simulink library "lib_controls"  (Simulink 7.9)
settings: Solver=ode45  SolverMode=SingleTasking  StartTime=0.0  StopTime=10.0  RelTol=1e-3
undefined symbols (not defined in the file or in its folder): amb_tmp, cs_charge_deplete_bool, cs_charge_pwr, cs_charge_trq, cs_clt_tmp, cs_decel_fc_off, cs_decel_regen_threshold, cs_dl_assist_trq_threshold, cs_dl_regen_trq_threshold, cs_electric_decel_spd, cs_electric_launch_spd, cs_electric_launch_spd_hi, cs_electric_launch_spd_lo, cs_eng_min_spd, cs_eng_on_soc, cs_fc_init_state, cs_fc_max_pwr_frac, cs_fc_min_pwr_frac, cs_fc_on, cs_fc_pwr_opt, cs_fc_spd_opt, cs_fuzzy_fuel_mode, cs_hi_soc, cs_hi_trq_frac, cs_lo_soc, cs_lo_trq_frac, cs_max_gc_spd, cs_max_pwr, cs_max_pwr_fall_rate, cs_max_pwr_rise_rate, cs_mc_assist_max_frac, cs_mc_assist_min_frac, cs_mc_assist_slope, cs_mc_regen_max_frac, cs_mc_regen_min_frac, cs_mc_regen_slope, cs_mean_eff, cs_mean_eff_bool, cs_min_gc_spd, cs_min_off_time, cs_min_pwr, cs_min_trq_frac, cs_mph_avg_time, cs_off_trq_frac, cs_plot_output, cs_pwr, cs_regen_avg_time, cs_scale_factor, cs_shutoff, cs_soc_range, cs_spd, cs_target_soc, cs_trq_to_soc_factor, cvt_locus_pwr, cvt_locus_spd, cyc_mph, enable_sim_stop_distance, enable_sim_stop_max_spd, enable_sim_stop_speed, enable_sim_stop_time ... (+110)
libraries: lib_controls x124, simulink3 x13, simulink x5, lib_etc x1
(part 14 of 17)

== system lib_controls/<vc> series/gearbox control for series  HV and EV/shifting1 ==
  gear number : Inport
  Constant : Constant  Value=gb_shift_delay-1e-6
  Relational Operator : RelationalOperator  Operator=<  InputSameDT=on
  time since last shift : Subsystem
      mask Display: disp('time since\nlast shift')
  out_1 : Outport  InitialOutput=0
  wires:
  Relational Operator/1 -> out_1/1
  gear number/1 -> time since last shift/1(in_1)
  Constant/1 -> Relational Operator/2
  time since last shift/1(out_1) -> Relational Operator/1

== system lib_controls/<vc> series/gearbox control for series  HV and EV/upshift  command ==
  prev gear number : Inport
  engine load : Inport  Port=2
  engine speed : Inport  Port=3
  Mux : Mux  Inputs=2
  Relational Operator : RelationalOperator  Operator=<  InputSameDT=on
  load fraction : Subsystem  mask(Gear Selector){spd=gb_upshift_spd, load=gb_upshift_load}
      mask prompts: spd "Speeds:"; load "Load Fractions:"
      mask help:
      | This block will perform a linear interplation (extrapolation outside of bounds) to determine the shift point load fraction associated with the current gear number and speed.
      |
      | The Speeds parameter should be defined as an array of vectors containing speeds for each gear number.  The Load Fractions parameter should be defined as a array of vectors containing load fractions indexed by the speeds in the Speeds parameter for each gear number.
      mask Help:
      | Reference the base workspace variables - gb_**shift_spd and gb_**shift_load  where ** is either up for upshift conditions or dn for downshift conditions.
      | 
      | Or define the arrays as follows:
      | 
      | {[spd1 spd2 spd3 spd4]; [spd1 spd2 spd3 spd4]; ...}
      | 
      | {[load1 load2 load3 load4]; [load1 load2 load3 load4]; ...}
      | 
      | where each array contains one row for each gear in the gearbox.  Speeds should be defined in rad/s and loads as a decimal fraction.
  command : Outport  InitialOutput=0
  wires:
  load fraction/1(Out1) -> Relational Operator/2
  engine load/1 -> Relational Operator/1
  prev gear number/1 -> Mux/1
  Mux/1 -> load fraction/1(In1)
  engine speed/1 -> Mux/2
  Relational Operator/1 -> command/1

== system lib_controls/<vc> series/motor controller logic/Block NOTES ==
  note: This block models a motor/controller's logic, modulating the power input requirement as follows:
      | - enforcing the maximum current limit of the motor/controller
      | - shutting the motor off if the average speed over the time step ==0
      | - shutting the motor off if the transmission is shifting.

== system lib_controls/<vc> series/motor controller logic/Sign ==
  in_1 : Inport
  Constant : Constant  Value=0
  Relational Operator : RelationalOperator  Operator=>  InputSameDT=on
  Relational Operator1 : RelationalOperator  Operator=<  InputSameDT=on
  Sum : Sum  Inputs=+-  SaturateOnIntegerOverflow=on  InputSameDT=on  OutDataTypeStr=Inherit: Same as first input
  out_1 : Outport  InitialOutput=0
  wires:
  Sum/1 -> out_1/1
  Relational Operator/1 -> Sum/1
  Relational Operator1/1 -> Sum/2
  Constant/1 -> Relational Operator/2, Relational Operator1/2
  in_1/1 -> Relational Operator1/1, Relational Operator/1

== system lib_controls/<vc> series/series 'clutch' control/Block NOTES ==
  note: There is no clutch, per se, in the series hybrid vehicle, that is connected to
      | the engine.  This clutch control is provided to tell the fuel converter (a.k.a. engine)
      | when it can spin up freely.  The fuel converter spins up or down when the 'clutch' is
      | disengaged, and provides torque when the 'clutch' is engaged (signal==3).
      |
      | Here, the fuel converter spins up when the engine has been off within the
      | past 0.5 s (or one time step, whichever is greater).  At all other times, the fuel
      | converter provides torque to the generator.

== system lib_controls/Adaptive control strategy <cs>/Delta SOC expected from regen/Subsystem ==
  in_1 : Inport
  1/average time : Constant  Value=1/n
  Integrator : Integrator
  Product : Product  SaturateOnIntegerOverflow=on  RndMeth=Zero  InputSameDT=on  OutDataTypeStr=Inherit: Same as first input
  Sum : Sum  Inputs=+-  SaturateOnIntegerOverflow=on  InputSameDT=on  OutDataTypeStr=Inherit: Same as first input
  Transport Delay : TransportDelay  DelayTime=n
  out_1 : Outport  InitialOutput=0
  wires:
  1/average time/1 -> Product/2
  Product/1 -> out_1/1
  in_1/1 -> Integrator/1
  Sum/1 -> Product/1
  Transport Delay/1 -> Sum/2
  Integrator/1 -> Transport Delay/1, Sum/1

== system lib_controls/Adaptive control strategy <cs>/Finds operation  point - energy/emissions  weighting/Minimize the  energy used  and emissions ==
  note: Note: acc_elec_pwr_est is placed
      | outside of Min. Energy/emis due to the fact
      | that it is a FROM block. FROM blocks cannot
      | be placed inside of enabled sub-systems
  input vector : Inport
  "  1" : Constant  Value=0
  Demux : Demux  Outputs=8
  Logical Operator : Logic  Operator=NOT  Inputs=1
  Min. Energy/emis : Subsystem  TreatAsAtomicUnit=on
  Zero T/w/spd case : Subsystem
  Zero Treq or wreq case : Switch  Threshold=eps  SaturateOnIntegerOverflow=on  InputSameDT=on
  total fuel used (gal)1 : ToWorkspace  VariableName=cs_Impact
  Tfc : Outport
  wires:
  Logical Operator/1 -> Min. Energy/emis/Enable
  Demux/8 -> Min. Energy/emis/8(ess_tmp)
  Min. Energy/emis/2(Impact) -> total fuel used (gal)1/1
  Zero Treq or wreq case/1 -> Tfc/1
  "  1"/1 -> Zero Treq or wreq case/1
  Min. Energy/emis/1(Tfc) -> Zero Treq or wreq case/3
  Demux/1 -> Zero T/w/spd case/1(Treq), Min. Energy/emis/1(Treq)
  Demux/2 -> Zero T/w/spd case/2(wreq), Min. Energy/emis/2(wreq)
  Demux/7 -> Min. Energy/emis/7(ex_cat_tmp)
  Demux/6 -> Min. Energy/emis/6(fc_clt_tmp)
  Demux/5 -> Min. Energy/emis/5(cyc_mph_r)
  Demux/4 -> Min. Energy/emis/4(SOC)
  Demux/3 -> Min. Energy/emis/3(DeltaSOC regen)
  input vector/1 -> Demux/1
  Zero T/w/spd case/1(zero req flag) -> Zero Treq or wreq case/2, Logical Operator/1
  [acc_elec_pwr_est] -> Min. Energy/emis/9(Elect Aux  Load Power)

== system lib_controls/Adaptive control strategy <cs>/Finds operation  point - energy/emissions  weighting/Subsystem ==
  in_1 : Inport
  1/average time : Constant  Value=1/n
  Integrator : Integrator
  Product : Product  SaturateOnIntegerOverflow=on  RndMeth=Zero  InputSameDT=on  OutDataTypeStr=Inherit: Same as first input
  Sum : Sum  Inputs=+-  SaturateOnIntegerOverflow=on  InputSameDT=on  OutDataTypeStr=Inherit: Same as first input
  Transport Delay : TransportDelay  DelayTime=n
  out_1 : Outport  InitialOutput=0
  wires:
  1/average time/1 -> Product/2
  Product/1 -> out_1/1
  in_1/1 -> Integrator/1
  Sum/1 -> Product/1
  Transport Delay/1 -> Sum/2
  Integrator/1 -> Transport Delay/1, Sum/1

== system lib_controls/Fuzzy Logic control strategy <cs>/Fuzzy logic Code/Block NOTES ==
  note: This block calls the Fuzzy Controller through the Matlab-Function module.
      | The Fuzzy Control algorithm is written in MATLAB script. This makes it easy
      | for the user to edit the fuzzy algorithm and make changes.
      |
      | For more information on Matlab-functions, please refer to the MATLAB help files.

== system lib_controls/Fuzzy Logic control strategy <cs>/Input Scaling/Block NOTES ==
  note: INPUT SCALING
  note: In this block, inputs to the Fuzzy Logic controller are computed. The Current torque demand on the ICE
      | and the SoC are input as 2 scaled variables to the fuzzy controller. Both inputs are scaled from 1 to 11.
      |
      | For SoC, a value of cs_lo_soc would correspond to 1 and a value of cs_hi_soc would correspond to 11,
      | linearly interpolating between them.
      |
      | For the ICE Torque, any torque demand less than the target ICE torque would scale from 1 to 6. Any torque
      | demand greater than the target ICE torque would scale from 6 to 11 (the 2 being piecewise linear).
      |
      | The target ICE torque is the x g/s fuel use line, (FUEL USE MODE), or the peak efficiency line
      | (EFFICIENCY MODE).

== system lib_controls/Fuzzy Logic control strategy <cs>/Output scaling/Block NOTES ==
  note: OUTPUT SCALING
      | This bock scales the outputs of the controller to match the size of the components.
      | The scaling affects the way control signal is fed into the actuators. The scaling is done based
      | on the membership functions of the Fuzzy Control block.
      |
      | Here:
      |  DELTA ALPHA is scaled from 1 to 11, 1 representing zero torque, 6 representing target Torque
      | and 11 representing Max ICE torque. (the 2 regions being piecewise linear).

== system lib_controls/Fuzzy Logic control strategy with Emissions <cs>/Fuzzy logic Code/Block NOTES ==
  note: This block calls the Fuzzy Controller through the Matlab-Function module.
      | The Fuzzy Control algorithm is written in MATLAB script. This makes it easy
      | for the user to edit the fuzzy algorithm and make changes.
      |
      | For more information on Matlab-functions, please refer to the MATLAB help files.

== system lib_controls/Fuzzy Logic control strategy with Emissions <cs>/Input Scaling/Block NOTES ==
  note: In this block, inputs to the Fuzzy Logic controller are computed. The Current torque demand on the ICE
      | and the SoC are input as 2 scaled variables to the fuzzy controller. Both inputs are scaled from 1 to 11.
      |
      | For SoC, a value of cs_lo_soc would correspond to 1 and a value of cs_hi_soc would correspond to 11,
      | linearly interpolating between them.
      |
      | For the ICE Torque, any torque demand less than the target ICE torque would scale from 1 to 6. Any torque
      | demand greater than the target ICE torque would scale from 6 to 11 (the 2 being piecewise linear).
  note: INPUT SCALING
  note: TARGET TORQUE COMPUTATION
  note: The target (optimal) torque for a particular speed requested from the ICE is calculated using a weighted average of
      | the efficiency and emissions data for a particular speed in consideration.
      |
      | The calculation of the target torque involves calculating the minimum of a cost function. The competing quantities
      | of the cost function include the emissions and fuel economy for all torques at that speed, weighed by their
      | respective weights.
      |
      | The relative importance for the competing quantities (weights) are changed during the simulation,
      | to reflect changes in driving conditions. For example, during a cold start, emissions are given higher priority. Also,
      | if the electric motor has been reaching it's maximum assist capability in the wake of the torque request not being met,
      | then emissions are sacrificed for higher torque from the ICE.

== system lib_controls/Fuzzy Logic control strategy with Emissions <cs>/Output scaling/Block NOTES ==
  note: OUTPUT SCALING
      | This bock scales the outputs of the controller to match the size of the components.
      | The scaling affects the way control signal is fed into the actuators. The scaling is done based
      | on the membership functions of the Fuzzy Control block.
      |
      | Here:
      |  DELTA ALPHA is scaled from 1 to 11, 1 representing zero torque, 6 representing target Torque
      | and 11 representing Max ICE torque. (the 2 regions being piecewise linear).

== system lib_controls/Fuzzy Logic control strategy with Emissions <cs>/SoC /Block NOTES ==
  note: This block scales the battery SOC so as to feed it into the Fuzzy controller.
      | 1 represents the lower limit of allowable battery SOC while 11 represents the higher
      | limit of allowable battery SOC.

== system lib_controls/Insight electric assist control strategy <cs> DIRECT SPLIT/Alternator Function/Block NOTES ==
  note: ALTERNATOR FUNCTION
      | In the HONDA Insight, there is no separate alternator for the vehicle in the powertrain
      | to supply power for the accessory loads. The main electric motor is the alternator for the vehicle.
      | Thus, it always produces a small negative torque for driving the accessory loads.  But the electric
      | motor has to take into account, the component efficiencies, and thus, is forced
      | to regenerate a little more than the accessory load.
      |
      | During assist, the battery pack supplies the electrical accessory loads.

== system lib_controls/Insight electric assist control strategy <cs> DIRECT SPLIT/SoC Correction/Block NOTES ==
  note: HONDA INSIGHT SoC Correction STRATEGY
      |
      | In the HONDA Insight strategy, the electric motor assist is independent on the SoC of the battery pack
      | except at low and high SoCs. (Based on test results).
      |
      | At high SoCs, above 0.8, all regeneration (charging) is stopped. At low SoCs, below 0.35 (approx),
      | the assist capacity of the motor is limited, and all assist is cut off below an SoC of 0.2.

== system lib_controls/SubSystem/braking strategy/Block NOTES ==
  note: This controller determines how much braking
      | force the front and rear  friction brakes will supply.

== system lib_controls/SubSystem/front and rear brake controller (achievable)/Block NOTES ==
  note: This block apportions required friction braking force between the
      | front (drive) and rear brakes.  Vehicle speed for brake strategy is
      | computed assuming zero slip.

== system lib_controls/SubSystem/front and rear brake controller (achievable)/braking force supplied by front friction brakes (N) ==
  add'l braking force req'd (N) : Inport
  possible speed (mph) : Inport  Port=2
  max front brake force (N) : Inport  Port=3
  Block NOTES : Subsystem
      mask Display: disp('Block\nNOTES')
  Constant : Constant  Value=1+eps
  Constant1 : Constant  Value=0.6
  Keep 0<frac<1 : Saturate  UpperLimit=1  LowerLimit=0
  MinMax : MinMax  Function=max  Inputs=2  SaturateOnIntegerOverflow=on  InputSameDT=on
  Product : Product  Inputs=**  SaturateOnIntegerOverflow=on  RndMeth=Zero  InputSameDT=on  OutDataTypeStr=Inherit: Same as first input
  Product1 : Product  Inputs=*/  SaturateOnIntegerOverflow=on  RndMeth=Zero  InputSameDT=on  OutDataTypeStr=Inherit: Same as first input
  Saturation : Saturate  UpperLimit=max(wh_fa_fric_brake_mph)  LowerLimit=min(wh_fa_fric_brake_mph)
  Saturation1 : Saturate  UpperLimit=max(wh_fa_dl_brake_mph)  LowerLimit=min(wh_fa_dl_brake_mph)
  Sum : Sum  Inputs=-+  SaturateOnIntegerOverflow=on  InputSameDT=on  OutDataTypeStr=Inherit: Same as first input
  Switch1 : Switch  Threshold=eps  SaturateOnIntegerOverflow=on  InputSameDT=on
  driveline braking fraction : Lookup  InputValues=wh_fa_dl_brake_mph  Table=wh_fa_dl_brake_frac  SaturateOnIntegerOverflow=on
  front friction braking fraction : Lookup  InputValues=wh_fa_fric_brake_mph  Table=wh_fa_fric_brake_frac  SaturateOnIntegerOverflow=on
  braking force from front-axle friction brakes (N) : Outport  InitialOutput=0
  wires:
  Keep 0<frac<1/1 -> Product/2
  Switch1/1 -> Keep 0<frac<1/1
  MinMax/1 -> braking force from front-axle friction brakes (N)/1
  Product/1 -> MinMax/1
  max front brake force (N)/1 -> MinMax/2
  add'l braking force req'd (N)/1 -> Product/1
  Constant/1 -> Sum/2
  driveline braking fraction/1 -> Sum/1
  front friction braking fraction/1 -> Product1/1
  Product1/1 -> Switch1/1
  Sum/1 -> Product1/2, Switch1/2
  Constant1/1 -> Switch1/3
  Saturation/1 -> front friction braking fraction/1
  Saturation1/1 -> driveline braking fraction/1
  possible speed (mph)/1 -> Saturation1/1, Saturation/1

== system lib_controls/SubSystem/shifting/time since last shift ==
  in_1 : Inport
  just shifted : Subsystem
      mask Display: disp('just\nshifted')
  timer : Subsystem
      mask Display: disp('timer')
  out_1 : Outport  InitialOutput=0
  wires:
  in_1/1 -> just shifted/1(in_1)
  just shifted/1(out_1) -> timer/1(trigger)
  timer/1(time) -> out_1/1

== system lib_controls/SubSystem/sim stop subsystem/Block NOTES ==
  note: This block controls the simulation stop time.  The simulation maybe
      | stop based on the achievement of a specified speed, a max speed, a time, a distance, or an engine condition.

== system lib_controls/SubSystem/sim stop subsystem/stop sim distance ==
  distance : Inport
  Enable : EnablePort
  Const : Constant  Value=sim_stop_distance
  Relational Operator2 : RelationalOperator  Operator=>  InputSameDT=on
  Out1 : Outport  InitialOutput=0
  wires:
  distance/1 -> Relational Operator2/1
  Const/1 -> Relational Operator2/2
  Relational Operator2/1 -> Out1/1

== system lib_controls/SubSystem/sim stop subsystem/stop sim fc ==
  engine on? : Inport
  Enable : EnablePort
  Clock : Clock
  Const : Constant  Value=j17_endtimes
  Logical Operator : Logic
  Logical Operator1 : Logic  Operator=OR
  Logical Operator2 : Logic  Operator=OR  Inputs=1
  Manual Switch : simulink3/Nonlinear/Manual Switch  sw=0  action=0
  Memory : Memory
  Relational Operator : RelationalOperator  Operator===  InputSameDT=on
  Relational Operator1 : RelationalOperator  InputSameDT=on
  Out1 : Outport  InitialOutput=0
  wires:
  Manual Switch/1 -> Logical Operator2/1
  Relational Operator1/1 -> Manual Switch/2
  Relational Operator/1 -> Manual Switch/1
  Clock/1 -> Relational Operator1/1, Relational Operator/1
  Const/1 -> Relational Operator1/2, Relational Operator/2
  engine on?/1 -> Logical Operator1/1
  Memory/1 -> Logical Operator1/2
  Logical Operator1/1 -> Memory/1, Logical Operator/1
  Logical Operator2/1 -> Logical Operator/2
  Logical Operator/1 -> Out1/1

== system lib_controls/SubSystem/sim stop subsystem/stop sim max spd ==
  speed : Inport
  Enable : EnablePort
  Block NOTES : Subsystem
      mask Display: disp('Block\nNOTES')
  Const : Constant  Value=eps
  Logical Operator : Logic
  Relational Operator2 : RelationalOperator  Operator=>  InputSameDT=on
  Relational Operator3 : RelationalOperator  Operator=<=  InputSameDT=on
  Transport Delay : TransportDelay  DelayTime=(gb_shift_delay*5)+1
  Out1 : Outport  InitialOutput=0
  wires:
  Const/1 -> Relational Operator2/2
  Relational Operator2/1 -> Logical Operator/2
  Logical Operator/1 -> Out1/1
  speed/1 -> Relational Operator3/1, Relational Operator2/1, Transport Delay/1
  Transport Delay/1 -> Relational Operator3/2
  Relational Operator3/1 -> Logical Operator/1

== system lib_controls/SubSystem/sim stop subsystem/stop sim speed ==
  speed : Inport
  Enable : EnablePort
  Const : Constant  Value=sim_stop_speed
  Relational Operator2 : RelationalOperator  Operator=>  InputSameDT=on
  Out1 : Outport  InitialOutput=0
  wires:
  Relational Operator2/1 -> Out1/1
  Const/1 -> Relational Operator2/2
  speed/1 -> Relational Operator2/1

== system lib_controls/SubSystem/sim stop subsystem/stop sim time ==
  time : Inport
  Enable : EnablePort
  Const : Constant  Value=sim_stop_time
  Relational Operator2 : RelationalOperator  Operator=>  InputSameDT=on
  Out1 : Outport  InitialOutput=0
  wires:
  time/1 -> Relational Operator2/1
  Const/1 -> Relational Operator2/2
  Relational Operator2/1 -> Out1/1

== system lib_controls/SubSystem/traction control/Block NOTES ==
  note: Requested speed and force are limited by the
      | tractive characteristics of the tires in this block.

== system lib_controls/SubSystem/traction control/apply tire traction limit to req'd speed (m/s) ==
  "requested time-step  average vehicle speed (m/s) " : Inport
  vehicle speed at beginning of time step (m/s) : Inport  Port=2
  Block NOTES : Subsystem
      mask Display: disp('Block\nNOTES')
  Clock : Clock
  Constant : Constant  Value=veh_gravity
  Constant1 : Constant  Value=0.5*veh_gravity*wh_2nd_rrc
  Constant10 : Constant  Value=veh_gravity
  Constant11 : Constant  Value=wh_1st_rrc
  Constant2 : Constant  Value=max(wh_slip_force_coeff)*veh_gravity*veh_front_wt_frac
  Constant3 : Constant  Value=0.125*veh_air_density*veh_CD*veh_FA
  Constant4 : Constant  Value=max(wh_slip_force_coeff)*veh_cg_height/veh_wheelbase
  Constant6 : Constant  Value=0.375*veh_air_density*veh_CD*veh_FA
  Constant7 : Constant  Value=0.5*veh_gravity*wh_2nd_rrc
  Constant9 : Constant  Value=max(wh_slip_force_coeff)*veh_cg_height/veh_wheelbase
  Fcn : Fcn  Expr=1/u
  Memory : Memory  X0=-0.1
  MinMax : MinMax  Inputs=2  SaturateOnIntegerOverflow=on  InputSameDT=on
  Product : Product  Inputs=4  SaturateOnIntegerOverflow=on  RndMeth=Zero  InputSameDT=on  OutDataTypeStr=Inherit: Same as first input
  Product{1,3,6..7,9..11} (7 alike) : Product  Inputs=3  SaturateOnIntegerOverflow=on  RndMeth=Zero  InputSameDT=on  OutDataTypeStr=Inherit: Same as first input
  Product2 : Product  Inputs=4  SaturateOnIntegerOverflow=on  RndMeth=Zero  InputSameDT=on  OutDataTypeStr=Inherit: Same as first input
  Product4 : Product  SaturateOnIntegerOverflow=on  RndMeth=Zero  InputSameDT=on  OutDataTypeStr=Inherit: Same as first input
  Product5 : Product  SaturateOnIntegerOverflow=on  RndMeth=Zero  InputSameDT=on  OutDataTypeStr=Inherit: Same as first input
  Product8 : Product  SaturateOnIntegerOverflow=on  RndMeth=Zero  InputSameDT=on  OutDataTypeStr=Inherit: Same as first input
  Sum : Sum  Inputs=+---+-+  SaturateOnIntegerOverflow=on  InputSameDT=on  OutDataTypeStr=Inherit: Same as first input
  Sum1 : Sum  Inputs=+-  SaturateOnIntegerOverflow=on  InputSameDT=on  OutDataTypeStr=Inherit: Same as first input
  Sum2 : Sum  Inputs=++++  SaturateOnIntegerOverflow=on  InputSameDT=on  OutDataTypeStr=Inherit: Same as first input
  Sum3 : Sum  Inputs=-----+  SaturateOnIntegerOverflow=on  InputSameDT=on  OutDataTypeStr=Inherit: Same as first input
  Sum4 : Sum  SaturateOnIntegerOverflow=on  InputSameDT=on  OutDataTypeStr=Inherit: Same as first input
  Sum5 : Sum  SaturateOnIntegerOverflow=on  InputSameDT=on  OutDataTypeStr=Inherit: Same as first input
  Sum6 : Sum  SaturateOnIntegerOverflow=on  InputSameDT=on  OutDataTypeStr=Inherit: Same as first input
  Sum7 : Sum  Inputs=+++-  SaturateOnIntegerOverflow=on  InputSameDT=on  OutDataTypeStr=Inherit: Same as first input
  Trig Fn4 : Trigonometry  Operator=cos
  Trig Fn : Trigonometry  Operator=atan
  Trig Fn1 : Trigonometry
  current veh mass (kg){,1..7} (8 alike) : lib_controls/SubSystem/current veh mass (kg)
      settings: RTWFcnNameOpts=Auto  RTWFileNameOpts=Auto
  max speed at END of time step given tire traction limit (m/s) : Subsystem
      mask Display: disp('/')
  max time-step average speed (m/s) : Gain  Gain=0.5  SaturateOnIntegerOverflow=on  OutDataTypeStr=Inherit: Same as input  ParamDataTypeStr=Inherit: Same as input
  min speed at END of time step given tire traction limit (m/s) : Subsystem
      mask Display: disp('/')
  min time-step average speed (m/s) : Gain  Gain=0.5  SaturateOnIntegerOverflow=on  OutDataTypeStr=Inherit: Same as input  ParamDataTypeStr=Inherit: Same as input
  requested time-step average speed limited by tire traction (m/s) : MinMax  Function=max  Inputs=2  SaturateOnIntegerOverflow=on  InputSameDT=on
  out_1 : Outport  InitialOutput=0
  wires:
  current veh mass (kg)7/1 -> Product6/3
  current veh mass (kg)5/1 -> Product7/3
  current veh mass (kg)3/1 -> Product2/4
  current veh mass (kg)2/1 -> Product9/3
  current veh mass (kg)1/1 -> Product/4
  current veh mass (kg)/1 -> Product11/3
  Constant/1 -> Product11/1
  Product11/1 -> Sum3/2, Sum/2
  Sum6/1 -> Product11/2
  Trig Fn1/1 -> Product10/3, Sum6/2
  Constant10/1 -> Product10/2
  Constant4/1 -> Product10/1, Product2/1
  Product10/1 -> Sum/6
  Product3/1 -> Sum/7, Sum3/6
  current veh mass (kg)4/1 -> Product3/2
  max time-step average speed (m/s)/1 -> MinMax/2
  "requested time-step  average vehicle speed (m/s) "/1 -> MinMax/1
  Sum5/1 -> max time-step average speed (m/s)/1
  Constant2/1 -> Product9/1
  Constant11/1 -> Product8/1
  Product8/1 -> Sum6/1
  Trig Fn4/1 -> Product9/2, Product8/2, Product/3, Product7/2
  Clock/1 -> Memory/1, Sum1/1
  Sum1/1 -> Fcn/1
  Memory/1 -> Sum1/2
  current veh mass (kg)6/1 -> Product5/1
  Sum2/1 -> max speed at END of time step given tire traction limit (m/s)/2(in_2)
  min time-step average speed (m/s)/1 -> requested time-step average speed limited by tire traction (m/s)/2
  requested time-step average speed limited by tire traction (m/s)/1 -> out_1/1
  Sum4/1 -> min time-step average speed (m/s)/1
  min speed at END of time step given tire traction limit (m/s)/1(out_1) -> Sum4/1
  MinMax/1 -> requested time-step average speed limited by tire traction (m/s)/1
  Sum3/1 -> min speed at END of time step given tire traction limit (m/s)/1(in_1)
  Sum7/1 -> min speed at END of time step given tire traction limit (m/s)/2(in_2)
  Constant7/1 -> Product7/1
  Constant9/1 -> Product6/1
  Constant6/1 -> Product4/2
  Product4/1 -> Sum2/1, Sum7/1
  Product7/1 -> Sum2/2, Sum7/2
  Product5/1 -> Sum2/3, Sum7/3
  Product6/1 -> Sum2/4, Sum7/4
  Trig Fn/1 -> Trig Fn4/1, Trig Fn1/1
  vehicle speed at beginning of time step (m/s)/1 -> Sum5/2, Sum4/2, Product4/1, Product3/1, Product2/2, Product1/3, Product1/2, Product/2
  [grade] -> Trig Fn/1
  max speed at END of time step given tire traction limit (m/s)/1(out_1) -> Sum5/1
  Product2/1 -> Sum3/5, Sum/5
  Product9/1 -> Sum3/1, Sum/1
  Product/1 -> Sum3/3, Sum/3
  Product1/1 -> Sum3/4, Sum/4
  Sum/1 -> max speed at END of time step given tire traction limit (m/s)/1(in_1)
  Fcn/1 -> Product6/2, Product5/2, Product3/3, Product2/3
  Constant3/1 -> Product1/1
  Constant1/1 -> Product/1

== system lib_controls/SubSystem/traction control/enforce max.  front axle tractive force  due to slip (N) ==
  tractive force req'd at tire/road interface (N) : Inport
  requested time-step average vehicle speed (m/s) : Inport  Port=2
  speed at beginning of time step (m/s) : Inport  Port=3
  " " : MinMax  Inputs=2  SaturateOnIntegerOverflow=on  InputSameDT=on
  Block NOTES : Subsystem
      mask Display: disp('Block\nNOTES')
  Clock : Clock
  Constant : Constant  Value=veh_cg_height/veh_wheelbase
  Constant1 : Constant  Value=veh_gravity*veh_front_wt_frac
  Constant2 : Constant  Value=max(wh_slip_force_coeff)
  Gain : Gain  Gain=-1  SaturateOnIntegerOverflow=on  OutDataTypeStr=Inherit: Same as input  ParamDataTypeStr=Inherit: Same as input
  Gain1 : Gain  Gain=2  SaturateOnIntegerOverflow=on  OutDataTypeStr=Inherit: Same as input  ParamDataTypeStr=Inherit: Same as input
  Gain2 : Gain  Gain=veh_gravity  SaturateOnIntegerOverflow=on  OutDataTypeStr=Inherit: Same as input  ParamDataTypeStr=Inherit: Same as input
  Memory1 : Memory  X0=-0.1
  Product : Product  Inputs=*/  SaturateOnIntegerOverflow=on  RndMeth=Zero  InputSameDT=on  OutDataTypeStr=Inherit: Same as first input
  Product1 : Product  Inputs=3  SaturateOnIntegerOverflow=on  RndMeth=Zero  InputSameDT=on  OutDataTypeStr=Inherit: Same as first input
  Product2 : Product  SaturateOnIntegerOverflow=on  RndMeth=Zero  InputSameDT=on  OutDataTypeStr=Inherit: Same as first input
  Product3 : Product  Inputs=3  SaturateOnIntegerOverflow=on  RndMeth=Zero  InputSameDT=on  OutDataTypeStr=Inherit: Same as first input
  Sum : Sum  Inputs=+-  SaturateOnIntegerOverflow=on  InputSameDT=on  OutDataTypeStr=Inherit: Same as first input
  Sum1 : Sum  Inputs=+-  SaturateOnIntegerOverflow=on  InputSameDT=on  OutDataTypeStr=Inherit: Same as first input
  Sum2 : Sum  SaturateOnIntegerOverflow=on  InputSameDT=on  OutDataTypeStr=Inherit: Same as first input
  Trig Fn : Trigonometry  Operator=atan
  Trig Fn1 : Trigonometry
  Trig Fn2 : Trigonometry  Operator=cos
  current veh mass (kg) : lib_controls/SubSystem/current veh mass (kg)
      settings: RTWFcnNameOpts=Auto  RTWFileNameOpts=Auto
  tractive force request limited by slip-threshhold force (N)1 : MinMax  Function=max  Inputs=2  SaturateOnIntegerOverflow=on  InputSameDT=on
  weight on front axle (N) : Sum  Inputs=-+  SaturateOnIntegerOverflow=on  InputSameDT=on  OutDataTypeStr=Inherit: Same as first input
  slip-limited force (N) : Outport  InitialOutput=0
  weight on front axle (N)1 : Outport  Port=2  InitialOutput=0
  wires:
  current veh mass (kg)/1 -> Product1/3, Product3/1
  Trig Fn2/1 -> Product3/2
  Constant1/1 -> Product3/3
  Product3/1 -> weight on front axle (N)/2
  Trig Fn/1 -> Trig Fn2/1, Trig Fn1/1
  Gain2/1 -> Sum2/2
  Trig Fn1/1 -> Gain2/1
  [grade] -> Trig Fn/1
  Sum2/1 -> Product1/2
  Gain1/1 -> Sum2/1
  tractive force request limited by slip-threshhold force (N)1/1 -> slip-limited force (N)/1
  " "/1 -> tractive force request limited by slip-threshhold force (N)1/1
  Product2/1 -> Gain/1, " "/1
  tractive force req'd at tire/road interface (N)/1 -> " "/2
  Constant2/1 -> Product2/2
  Gain/1 -> tractive force request limited by slip-threshhold force (N)1/2
  Product/1 -> Gain1/1
  Sum1/1 -> Product/2
  Memory1/1 -> Sum1/2
  Clock/1 -> Memory1/1, Sum1/1
  Sum/1 -> Product/1
  speed at beginning of time step (m/s)/1 -> Sum/2
  requested time-step average vehicle speed (m/s)/1 -> Sum/1
  weight on front axle (N)/1 -> weight on front axle (N)1/1, Product2/1
  Constant/1 -> Product1/1
  Product1/1 -> weight on front axle (N)/1

== system lib_controls/SubSystem/traction control 2 axle/Block NOTES ==
  note: Requested speed and force are limited by the
      | tractive characteristics of the tires in this block.

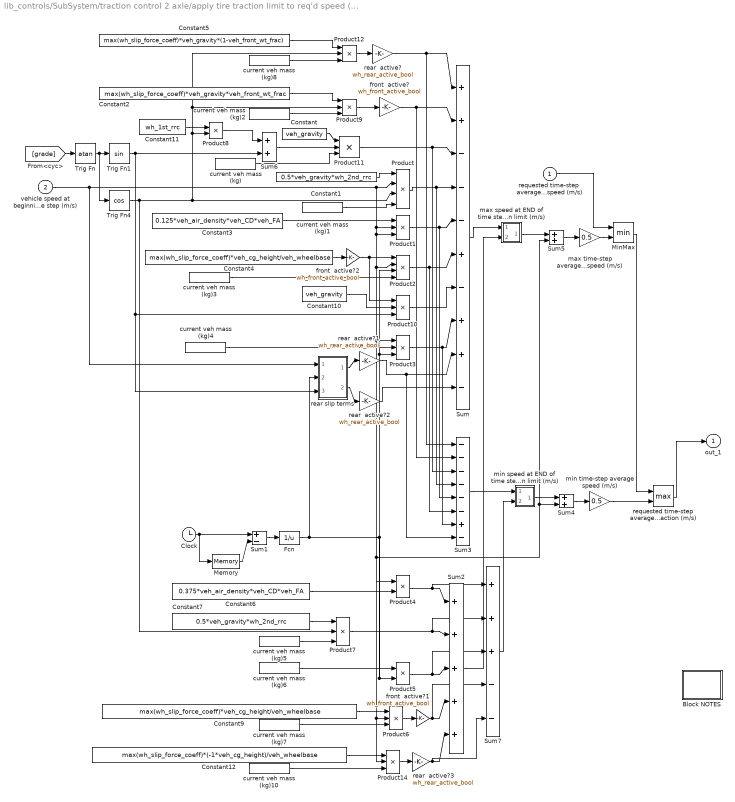
== system lib_controls/SubSystem/traction control 2 axle/apply tire traction limit to req'd speed (m/s) ==
  "requested time-step  average vehicle speed (m/s) " : Inport
  vehicle speed at beginning of time step (m/s) : Inport  Port=2
  Block NOTES : Subsystem
      mask Display: disp('Block\nNOTES')
  Clock : Clock
  Constant : Constant  Value=veh_gravity
  Constant1 : Constant  Value=0.5*veh_gravity*wh_2nd_rrc
  Constant10 : Constant  Value=veh_gravity
  Constant11 : Constant  Value=wh_1st_rrc
  Constant12 : Constant  Value=max(wh_slip_force_coeff)*(-1*veh_cg_height)/veh_wheelbase
  Constant2 : Constant  Value=max(wh_slip_force_coeff)*veh_gravity*veh_front_wt_frac
  Constant3 : Constant  Value=0.125*veh_air_density*veh_CD*veh_FA
  Constant4 : Constant  Value=max(wh_slip_force_coeff)*veh_cg_height/veh_wheelbase
  Constant5 : Constant  Value=max(wh_slip_force_coeff)*veh_gravity*(1-veh_front_wt_frac)
  Constant6 : Constant  Value=0.375*veh_air_density*veh_CD*veh_FA
  Constant7 : Constant  Value=0.5*veh_gravity*wh_2nd_rrc
  Constant9 : Constant  Value=max(wh_slip_force_coeff)*veh_cg_height/veh_wheelbase
  Fcn : Fcn  Expr=1/u
  Memory : Memory  X0=-0.1
  MinMax : MinMax  Inputs=2  SaturateOnIntegerOverflow=on  InputSameDT=on
  Product : Product  Inputs=4  SaturateOnIntegerOverflow=on  RndMeth=Zero  InputSameDT=on  OutDataTypeStr=Inherit: Same as first input
  Product{1,3,6..7,9..12,14} (9 alike) : Product  Inputs=3  SaturateOnIntegerOverflow=on  RndMeth=Zero  InputSameDT=on  OutDataTypeStr=Inherit: Same as first input
  Product2 : Product  Inputs=4  SaturateOnIntegerOverflow=on  RndMeth=Zero  InputSameDT=on  OutDataTypeStr=Inherit: Same as first input
  Product4 : Product  SaturateOnIntegerOverflow=on  RndMeth=Zero  InputSameDT=on  OutDataTypeStr=Inherit: Same as first input
  Product5 : Product  SaturateOnIntegerOverflow=on  RndMeth=Zero  InputSameDT=on  OutDataTypeStr=Inherit: Same as first input
  Product8 : Product  SaturateOnIntegerOverflow=on  RndMeth=Zero  InputSameDT=on  OutDataTypeStr=Inherit: Same as first input
  Sum : Sum  Inputs=++---+-++-  SaturateOnIntegerOverflow=on  InputSameDT=on  OutDataTypeStr=Inherit: Same as first input
  Sum1 : Sum  Inputs=+-  SaturateOnIntegerOverflow=on  InputSameDT=on  OutDataTypeStr=Inherit: Same as first input
  Sum2 : Sum  Inputs=+++++  SaturateOnIntegerOverflow=on  InputSameDT=on  OutDataTypeStr=Inherit: Same as first input
  Sum3 : Sum  Inputs=------+-  SaturateOnIntegerOverflow=on  InputSameDT=on  OutDataTypeStr=Inherit: Same as first input
  Sum4 : Sum  SaturateOnIntegerOverflow=on  InputSameDT=on  OutDataTypeStr=Inherit: Same as first input
  Sum5 : Sum  SaturateOnIntegerOverflow=on  InputSameDT=on  OutDataTypeStr=Inherit: Same as first input
  Sum6 : Sum  SaturateOnIntegerOverflow=on  InputSameDT=on  OutDataTypeStr=Inherit: Same as first input
  Sum7 : Sum  Inputs=+++--  SaturateOnIntegerOverflow=on  InputSameDT=on  OutDataTypeStr=Inherit: Same as first input
  Trig Fn4 : Trigonometry  Operator=cos
  Trig Fn : Trigonometry  Operator=atan
  Trig Fn1 : Trigonometry
  current veh mass (kg){,1..8,10} (10 alike) : lib_controls/SubSystem/current veh mass (kg)
      settings: RTWFcnNameOpts=Auto  RTWFileNameOpts=Auto
  front  active? : Gain  Gain=wh_front_active_bool  SaturateOnIntegerOverflow=on  OutDataTypeStr=Inherit: Same as input  ParamDataTypeStr=Inherit: Same as input
  front  active?1 : Gain  Gain=wh_front_active_bool  SaturateOnIntegerOverflow=on  OutDataTypeStr=Inherit: Same as input  ParamDataTypeStr=Inherit: Same as input
  front  active?2 : Gain  Gain=wh_front_active_bool  SaturateOnIntegerOverflow=on  OutDataTypeStr=Inherit: Same as input  ParamDataTypeStr=Inherit: Same as input
  max speed at END of time step given tire traction limit (m/s) : Subsystem
      mask Display: disp('/')
  max time-step average speed (m/s) : Gain  Gain=0.5  SaturateOnIntegerOverflow=on  OutDataTypeStr=Inherit: Same as input  ParamDataTypeStr=Inherit: Same as input
  min speed at END of time step given tire traction limit (m/s) : Subsystem
      mask Display: disp('/')
  min time-step average speed (m/s) : Gain  Gain=0.5  SaturateOnIntegerOverflow=on  OutDataTypeStr=Inherit: Same as input  ParamDataTypeStr=Inherit: Same as input
  rear  active?{,1..3} (4 alike) : Gain  Gain=wh_rear_active_bool  SaturateOnIntegerOverflow=on  OutDataTypeStr=Inherit: Same as input  ParamDataTypeStr=Inherit: Same as input
  rear slip terms : Subsystem
  requested time-step average speed limited by tire traction (m/s) : MinMax  Function=max  Inputs=2  SaturateOnIntegerOverflow=on  InputSameDT=on
  out_1 : Outport  InitialOutput=0
  wires:
  Constant1/1 -> Product/1
  Constant3/1 -> Product1/1
  Fcn/1 -> Product2/3, Product3/3, Product5/2, Product6/2, Product14/2, rear slip terms/2(1/dt)
  Sum/1 -> max speed at END of time step given tire traction limit (m/s)/1(in_1)
  Product1/1 -> Sum/5, Sum3/5
  Product/1 -> Sum/4, Sum3/4
  Product9/1 -> front  active?/1
  Product2/1 -> Sum/6, Sum3/6
  max speed at END of time step given tire traction limit (m/s)/1(out_1) -> Sum5/1
  [grade] -> Trig Fn/1
  vehicle speed at beginning of time step (m/s)/1 -> Product/2, Product1/2, Product1/3, Product2/2, Product3/1, Product4/1, Sum4/2, Sum5/2, rear slip terms/1(initial speed)
  Trig Fn/1 -> Trig Fn1/1, Trig Fn4/1
  Product6/1 -> front  active?1/1
  Product5/1 -> Sum7/3, Sum2/3
  Product7/1 -> Sum7/2, Sum2/2
  Product4/1 -> Sum7/1, Sum2/1
  Constant6/1 -> Product4/2
  Constant9/1 -> Product6/1
  Constant7/1 -> Product7/1
  Sum7/1 -> min speed at END of time step given tire traction limit (m/s)/2(in_2)
  Sum3/1 -> min speed at END of time step given tire traction limit (m/s)/1(in_1)
  MinMax/1 -> requested time-step average speed limited by tire traction (m/s)/1
  min speed at END of time step given tire traction limit (m/s)/1(out_1) -> Sum4/1
  Sum4/1 -> min time-step average speed (m/s)/1
  requested time-step average speed limited by tire traction (m/s)/1 -> out_1/1
  min time-step average speed (m/s)/1 -> requested time-step average speed limited by tire traction (m/s)/2
  Sum2/1 -> max speed at END of time step given tire traction limit (m/s)/2(in_2)
  current veh mass (kg)6/1 -> Product5/1
  Memory/1 -> Sum1/2
  Sum1/1 -> Fcn/1
  Clock/1 -> Sum1/1, Memory/1
  Trig Fn4/1 -> Product7/2, Product/3, Product8/2, Product9/2, Product12/2
  Product8/1 -> Sum6/1
  Constant11/1 -> Product8/1
  Constant2/1 -> Product9/1
  Sum5/1 -> max time-step average speed (m/s)/1
  "requested time-step  average vehicle speed (m/s) "/1 -> MinMax/1
  max time-step average speed (m/s)/1 -> MinMax/2
  current veh mass (kg)4/1 -> Product3/2
  Product3/1 -> Sum/8, Sum3/7
  Product10/1 -> Sum/7
  Constant4/1 -> front  active?2/1
  Constant10/1 -> Product10/2
  Trig Fn1/1 -> Sum6/2, Product10/3, rear slip terms/3(sin(theta))
  Sum6/1 -> Product11/2
  Product11/1 -> Sum/3, Sum3/3
  Constant/1 -> Product11/1
  current veh mass (kg)/1 -> Product11/3
  current veh mass (kg)1/1 -> Product/4
  current veh mass (kg)2/1 -> Product9/3
  current veh mass (kg)3/1 -> Product2/4
  current veh mass (kg)5/1 -> Product7/3
  current veh mass (kg)7/1 -> Product6/3
  Product12/1 -> rear  active?/1
  Constant5/1 -> Product12/1
  current veh mass (kg)8/1 -> Product12/3
  rear  active?/1 -> Sum/1, Sum3/1
  rear slip terms/1(Out1) -> rear  active?1/1
  rear slip terms/2(Out2) -> rear  active?2/1
  Product14/1 -> rear  active?3/1
  Constant12/1 -> Product14/1
  current veh mass (kg)10/1 -> Product14/3
  rear  active?1/1 -> Sum/9, Sum3/8
  rear  active?2/1 -> Sum/10
  rear  active?3/1 -> Sum7/5, Sum2/5
  front  active?/1 -> Sum/2, Sum3/2
  front  active?1/1 -> Sum7/4, Sum2/4
  front  active?2/1 -> Product2/1, Product10/1

== system lib_controls/SubSystem/traction control 2 axle/enforce max.  front axle tractive force  due to slip (N) ==
  tractive force req'd at tire/road interface (N) : Inport
  requested time-step average vehicle speed (m/s) : Inport  Port=2
  speed at beginning of time step (m/s) : Inport  Port=3
  " " : MinMax  Inputs=2  SaturateOnIntegerOverflow=on  InputSameDT=on
  Block NOTES : Subsystem
      mask Display: disp('Block\nNOTES')
  Constant2 : Constant  Value=max(wh_slip_force_coeff)
  Gain : Gain  Gain=-1  SaturateOnIntegerOverflow=on  OutDataTypeStr=Inherit: Same as input  ParamDataTypeStr=Inherit: Same as input
  Product1 : Product  SaturateOnIntegerOverflow=on  RndMeth=Zero  InputSameDT=on  OutDataTypeStr=Inherit: Same as first input
  Product2 : Product  SaturateOnIntegerOverflow=on  RndMeth=Zero  InputSameDT=on  OutDataTypeStr=Inherit: Same as first input
  Product3 : Product  Inputs=*/  SaturateOnIntegerOverflow=on  RndMeth=Zero  InputSameDT=on  OutDataTypeStr=Inherit: Same as first input
  Product4 : Product  Inputs=*/  SaturateOnIntegerOverflow=on  RndMeth=Zero  InputSameDT=on  OutDataTypeStr=Inherit: Same as first input
  Sum1 : Sum  SaturateOnIntegerOverflow=on  InputSameDT=on  OutDataTypeStr=Inherit: Same as first input
  Sum2 : Sum  SaturateOnIntegerOverflow=on  InputSameDT=on  OutDataTypeStr=Inherit: Same as first input
  front : Subsystem
  front  active? : Gain  Gain=wh_front_active_bool  SaturateOnIntegerOverflow=on  OutDataTypeStr=Inherit: Same as input  ParamDataTypeStr=Inherit: Same as input
  front traction ratio : ToWorkspace  VariableName=front_traction_ratio_orig
  rear : Subsystem
  rear  active? : Gain  Gain=wh_rear_active_bool  SaturateOnIntegerOverflow=on  OutDataTypeStr=Inherit: Same as input  ParamDataTypeStr=Inherit: Same as input
  tractive force request limited by slip-threshhold force (N)1 : MinMax  Function=max  Inputs=2  SaturateOnIntegerOverflow=on  InputSameDT=on
  slip-limited force (N) : Outport  InitialOutput=0
  weight on front axle (N) : Outport  Port=2  InitialOutput=0
  weight on rear axle (N) : Outport  Port=3  InitialOutput=0
  front/total traction ratio : Outport  Port=4  InitialOutput=0
  wires:
  front/1(Out1) -> Product2/1, weight on front axle (N)/1
  requested time-step average vehicle speed (m/s)/1 -> front/1(In1), rear/1(In1)
  speed at beginning of time step (m/s)/1 -> front/2(In2), rear/2(In2)
  Gain/1 -> tractive force request limited by slip-threshhold force (N)1/2
  Constant2/1 -> Product2/2, Product1/2
  tractive force req'd at tire/road interface (N)/1 -> " "/2
  " "/1 -> tractive force request limited by slip-threshhold force (N)1/1
  tractive force request limited by slip-threshhold force (N)1/1 -> slip-limited force (N)/1
  rear/1(Out1) -> weight on rear axle (N)/1, Product1/1
  Sum1/1 -> " "/1, Gain/1, Product3/2
  Product1/1 -> rear  active?/1, Sum2/2
  Product2/1 -> front  active?/1, Sum2/1, Product4/1
  Product3/1 -> front/total traction ratio/1
  front  active?/1 -> Sum1/1, Product3/1
  rear  active?/1 -> Sum1/2
  Sum2/1 -> Product4/2
  Product4/1 -> front traction ratio/1

== system lib_controls/SubSystem/traction control J2452/Block NOTES ==
  note: Requested speed and force are limited by the
      | tractive characteristics of the tires in this block.

== system lib_controls/SubSystem/traction control J2452/apply tire traction limit to req'd speed (m/s) ==
  "requested time-step  average vehicle speed (m/s) " : Inport
  vehicle speed at beginning of time step (m/s) : Inport  Port=2
  Block NOTES : Subsystem
      mask Display: disp('Block\nNOTES')
  Clock : Clock
  Constant : Constant  Value=veh_CD
  Constant1 : Constant  Value=veh_FA
  Constant10 : Constant  Value=veh_gravity
  Constant11 : Constant  Value=(veh_cg_height/veh_wheelbase)
  Constant12 : Constant  Value=wh_radius
  Constant13 : Constant  Value=veh_front_wt_frac
  Constant14 : Constant  Value=0
  Constant2 : Constant  Value=max(wh_slip_force_coeff)*veh_gravity*veh_front_wt_frac
  Constant3 : Constant  Value=veh_air_density
  Constant4 : Constant  Value=veh_rr_alpha
  Constant5 : Constant  Value=veh_rr_beta
  Constant6 : Constant  Value=veh_rr_a
  Constant7 : Constant  Value=veh_rr_b
  Constant8 : Constant  Value=veh_rr_c
  Constant9 : Constant  Value=wh_pressure
  Curvature Correction Factor : Constant  Value=(veh_roadwheel_radius/(veh_roadwheel_radius+wh_radius))  VectorParams1D=off
  Error Check : MinMax  Function=max  Inputs=2  SaturateOnIntegerOverflow=on  InputSameDT=on
  Math Function3 : Math  Operator=sqrt  SaturateOnIntegerOverflow=on
  Memory : Memory  X0=-0.1
  Memory1 : Memory  X0=-0.1
  MinMax : MinMax  Inputs=2  SaturateOnIntegerOverflow=on  InputSameDT=on
  Mux : Mux  Inputs=17
  Product1 : Product  Inputs=3  SaturateOnIntegerOverflow=on  RndMeth=Zero  InputSameDT=on  OutDataTypeStr=Inherit: Same as first input
  Product{2..7} (6 alike) : Product  SaturateOnIntegerOverflow=on  RndMeth=Zero  InputSameDT=on  OutDataTypeStr=Inherit: Same as first input
  Product9 : Product  Inputs=3  SaturateOnIntegerOverflow=on  RndMeth=Zero  InputSameDT=on  OutDataTypeStr=Inherit: Same as first input
  Sum : Sum  Inputs=+-  SaturateOnIntegerOverflow=on  InputSameDT=on  OutDataTypeStr=Inherit: Same as first input
  Sum1 : Sum  Inputs=+-  SaturateOnIntegerOverflow=on  InputSameDT=on  OutDataTypeStr=Inherit: Same as first input
  Sum4 : Sum  Inputs=+-  SaturateOnIntegerOverflow=on  InputSameDT=on  OutDataTypeStr=Inherit: Same as first input
  Sum5 : Sum  Inputs=-+  SaturateOnIntegerOverflow=on  InputSameDT=on  OutDataTypeStr=Inherit: Same as first input
  Trig Fn : Trigonometry  Operator=atan
  Trig Fn1 : Trigonometry  Operator=cos
  Trig Fn2 : Trigonometry  Operator=atan
  Trig Fn3 : Trigonometry  Operator=atan
  Trig Fn4 : Trigonometry  Operator=cos
  Vf : Fcn  Expr=-1/2*(-2*u(4)*u(17)-2*u(1)*u(6)+4*u(13)^u(8)*u(6)*(1/2*u(15))^u(9)*u(10)+4*u(13)^u(8)*u(6)*(1/2*u(15))^u(9)*u(11)*u(17)+4*u(13)^u(8)*u(6)*(1/2*u(15))^u(9)*u(12)*u(17)^2+4*u(13)^u(8)*u(6)*(1/2*u(16))^u(9)*u(10)+4*u(13)^u(8)*u(6)*(1/2*u(16))^u(9)*u(11)*u(17)+4*u(13)^u(8)*u(6)*(1/2*u(16))^u(9)*u(12)*u(17)^2+u(7)*u(3)*u(5)*u(17)^2*u(6)+2*u(4)*u(14)*sin(u(2))*u(6))/u(4)
  current veh mass (kg)1 : lib_controls/SubSystem/current veh mass (kg)
      settings: RTWFcnNameOpts=Auto  RTWFileNameOpts=Auto
  current veh mass (kg)2 : lib_controls/SubSystem/current veh mass (kg)
      settings: RTWFcnNameOpts=Auto  RTWFileNameOpts=Auto
  current veh mass (kg)6 : lib_controls/SubSystem/current veh mass (kg)
      settings: RTWFcnNameOpts=Auto  RTWFileNameOpts=Auto
  unit conversion : Gain  Gain=3.6*3.6  SaturateOnIntegerOverflow=on  OutDataTypeStr=Inherit: Same as input  ParamDataTypeStr=Inherit: Same as input
  unit conversion2 : Gain  Gain=3.6  SaturateOnIntegerOverflow=on  OutDataTypeStr=Inherit: Same as input  ParamDataTypeStr=Inherit: Same as input
  out_1 : Outport  InitialOutput=0
  wires:
  Product7/1 -> unit conversion/1
  Constant8/1 -> Product7/2
  Product3/1 -> unit conversion2/1
  Constant7/1 -> Product3/2
  Product2/1 -> Mux/10
  Constant6/1 -> Product2/2
  Math Function3/1 -> Product7/1, Product3/1, Product2/1
  Curvature Correction Factor/1 -> Math Function3/1
  unit conversion/1 -> Mux/12
  unit conversion2/1 -> Mux/11
  Error Check/1 -> Sum5/1, Mux/15  "Nf"
  Constant14/1 -> Error Check/2
  Sum/1 -> Error Check/1  "Nf"
  Sum5/1 -> Mux/16  "Nr=W-Nf"
  Product6/1 -> Sum5/2  "W"
  Memory1/1 -> Product4/1
  [wh_trq_a] -> Memory1/1
  vehicle speed at beginning of time step (m/s)/1 -> Mux/17
  current veh mass (kg)1/1 -> Product6/2, Product1/3
  Constant13/1 -> Product1/2
  Trig Fn4/1 -> Product6/1, Product1/1
  Trig Fn3/1 -> Trig Fn4/1
  [grade] -> Trig Fn3/1
  Constant10/1 -> Mux/14
  Constant9/1 -> Mux/13
  Constant5/1 -> Mux/9
  Constant4/1 -> Mux/8
  Constant3/1 -> Mux/7
  Constant1/1 -> Mux/5
  current veh mass (kg)6/1 -> Mux/4
  Constant/1 -> Mux/3
  Mux/1 -> Vf/1
  Trig Fn1/1 -> Product9/2
  current veh mass (kg)2/1 -> Product9/3
  "requested time-step  average vehicle speed (m/s) "/1 -> MinMax/1
  Constant2/1 -> Product9/1
  Trig Fn/1 -> Trig Fn1/1
  [grade] -> Trig Fn/1
  Product9/1 -> Mux/1  "Ftract"
  Sum1/1 -> Mux/6  "dt"
  Clock/1 -> Memory/1, Sum1/1
  Memory/1 -> Sum1/2
  [grade] -> Trig Fn2/1
  Trig Fn2/1 -> Mux/2  "theta"
  Product1/1 -> Sum/1
  MinMax/1 -> out_1/1
  Constant12/1 -> Product4/2
  Product4/1 -> Sum4/1
  [Fr_out] -> Sum4/2
  Sum4/1 -> Product5/1
  Constant11/1 -> Product5/2
  Product5/1 -> Sum/2
  Vf/1 -> MinMax/2

== system lib_controls/SubSystem/traction control J2452/enforce max.  front axle tractive force  due to slip (N) ==
  tractive force req'd at tire/road interface (N) : Inport
  requested time-step average vehicle speed (m/s) : Inport  Port=2
  speed at beginning of time step (m/s) : Inport  Port=3
  " " : MinMax  Inputs=2  SaturateOnIntegerOverflow=on  InputSameDT=on
  Block NOTES : Subsystem
      mask Display: disp('Block\nNOTES')
  Clock : Clock
  Constant : Constant  Value=veh_cg_height/veh_wheelbase
  Constant1 : Constant  Value=veh_gravity*veh_front_wt_frac
  Constant2 : Constant  Value=max(wh_slip_force_coeff)
  Gain : Gain  Gain=-1  SaturateOnIntegerOverflow=on  OutDataTypeStr=Inherit: Same as input  ParamDataTypeStr=Inherit: Same as input
  Gain1 : Gain  Gain=2  SaturateOnIntegerOverflow=on  OutDataTypeStr=Inherit: Same as input  ParamDataTypeStr=Inherit: Same as input
  Gain2 : Gain  Gain=veh_gravity  SaturateOnIntegerOverflow=on  OutDataTypeStr=Inherit: Same as input  ParamDataTypeStr=Inherit: Same as input
  Memory1 : Memory  X0=-0.1
  Product : Product  Inputs=*/  SaturateOnIntegerOverflow=on  RndMeth=Zero  InputSameDT=on  OutDataTypeStr=Inherit: Same as first input
  Product1 : Product  Inputs=3  SaturateOnIntegerOverflow=on  RndMeth=Zero  InputSameDT=on  OutDataTypeStr=Inherit: Same as first input
  Product2 : Product  SaturateOnIntegerOverflow=on  RndMeth=Zero  InputSameDT=on  OutDataTypeStr=Inherit: Same as first input
  Product3 : Product  Inputs=3  SaturateOnIntegerOverflow=on  RndMeth=Zero  InputSameDT=on  OutDataTypeStr=Inherit: Same as first input
  Sum : Sum  Inputs=+-  SaturateOnIntegerOverflow=on  InputSameDT=on  OutDataTypeStr=Inherit: Same as first input
  Sum1 : Sum  Inputs=+-  SaturateOnIntegerOverflow=on  InputSameDT=on  OutDataTypeStr=Inherit: Same as first input
  Sum2 : Sum  SaturateOnIntegerOverflow=on  InputSameDT=on  OutDataTypeStr=Inherit: Same as first input
  Trig Fn : Trigonometry  Operator=atan
  Trig Fn1 : Trigonometry
  Trig Fn2 : Trigonometry  Operator=cos
  current veh mass (kg) : lib_controls/SubSystem/current veh mass (kg)
      settings: RTWFcnNameOpts=Auto  RTWFileNameOpts=Auto
  tractive force request limited by slip-threshhold force (N)1 : MinMax  Function=max  Inputs=2  SaturateOnIntegerOverflow=on  InputSameDT=on
  weight on front axle (N) : Sum  Inputs=-+  SaturateOnIntegerOverflow=on  InputSameDT=on  OutDataTypeStr=Inherit: Same as first input
  slip-limited force (N) : Outport  InitialOutput=0
  weight on front axle (N)1 : Outport  Port=2  InitialOutput=0
  wires:
  Product1/1 -> weight on front axle (N)/1
  Constant/1 -> Product1/1
  weight on front axle (N)/1 -> Product2/1, weight on front axle (N)1/1
  requested time-step average vehicle speed (m/s)/1 -> Sum/1
  speed at beginning of time step (m/s)/1 -> Sum/2
  Sum/1 -> Product/1
  Clock/1 -> Sum1/1, Memory1/1
  Memory1/1 -> Sum1/2
  Sum1/1 -> Product/2
  Product/1 -> Gain1/1
  Gain/1 -> tractive force request limited by slip-threshhold force (N)1/2
  Constant2/1 -> Product2/2
  tractive force req'd at tire/road interface (N)/1 -> " "/2
  Product2/1 -> " "/1, Gain/1
  " "/1 -> tractive force request limited by slip-threshhold force (N)1/1
  tractive force request limited by slip-threshhold force (N)1/1 -> slip-limited force (N)/1
  Gain1/1 -> Sum2/1
  Sum2/1 -> Product1/2
  [grade] -> Trig Fn/1
  Trig Fn1/1 -> Gain2/1
  Gain2/1 -> Sum2/2
  Trig Fn/1 -> Trig Fn1/1, Trig Fn2/1
  Product3/1 -> weight on front axle (N)/2
  Constant1/1 -> Product3/3
  Trig Fn2/1 -> Product3/2
  current veh mass (kg)/1 -> Product3/1, Product1/3

== system lib_controls/SubSystem/traction control J2452 2 axle/Block NOTES ==
  note: Requested speed and force are limited by the
      | tractive characteristics of the tires in this block.
